simulink model "mass_spring"  (R2019a)
settings: Solver=VariableStepAuto  StartTime=0.0  StopTime=100  RelTol=1e-3
settings Model: Creator=shyreckdc  LastModifiedBy=shyreckdc

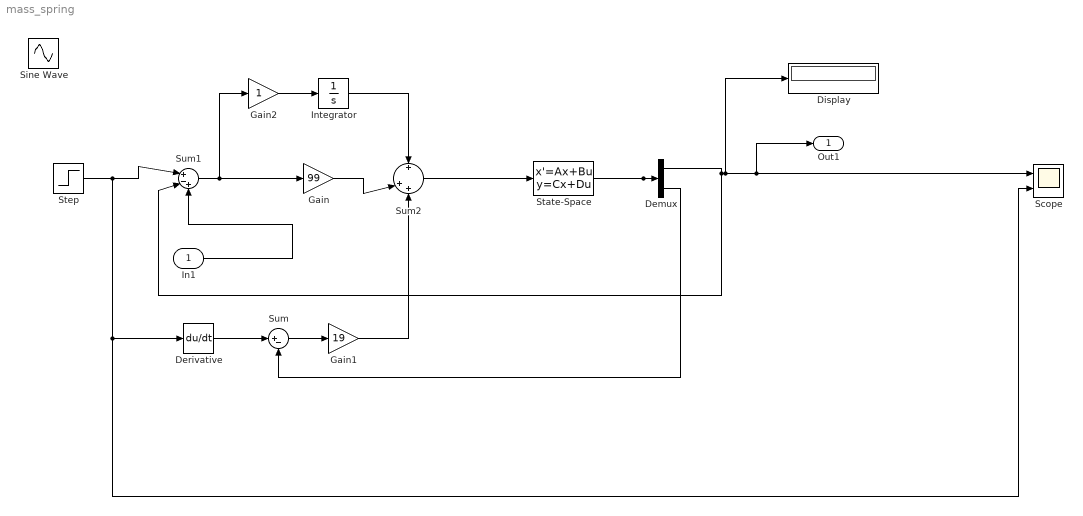
== system mass_spring ==
  In1 : Inport
  Demux : Demux  Outputs=2
  Derivative : Derivative
  Display : Display
  Gain : Gain  Gain=99
  Gain1 : Gain  Gain=19
  Gain2 : Gain
  Integrator : Integrator
  Scope : Scope  NumInputPorts=2
  Sine Wave : Sin  SampleTime=0
  State-Space : StateSpace  A=[0 1;-1 -1]  B=[0;1]  C=[1 0;0 1]  D=[0;0]  InitialCondition=[0;0]  ContinuousStateAttributes='position'
  Step : Step  Time=0  SampleTime=0
  Sum : Sum  Inputs=|+-
  Sum1 : Sum  Inputs=|+-+
  Sum2 : Sum  Inputs=+|++
  Out1 : Outport
  wires:
  State-Space/1 -> Demux/1
  Demux/2 -> Sum/2
  Demux/1 -> Display/1, Out1/1, Scope/1, Sum1/2
  Sum/1 -> Gain1/1
  Gain1/1 -> Sum2/3
  Gain/1 -> Sum2/2
  Sum2/1 -> State-Space/1
  Step/1 -> Scope/2, Derivative/1, Sum1/1
  In1/1 -> Sum1/3
  Sum1/1 -> Gain2/1, Gain/1
  Gain2/1 -> Integrator/1
  Derivative/1 -> Sum/1
  Integrator/1 -> Sum2/1
